simulink model "Vehicle_Model_999_Modular_roll_gradient"  (R2025b)
settings: Solver=ode23tb  StartTime=0.0  StopTime=30  MaxStep=0.001  RelTol=1e-3
values from neighbouring files (symbols this model uses):
  init_r = 0    [Run_this_first.m]
  init_vx = 0    [Run_this_first.m]
  init_vy = 0    [Run_this_first.m]
  Ki_array = zeros(size(Vx_array))    [Torque_vectoring_lookup_table_v3.m]    (also in Torque_vectoring_workspace_lookuptable_v2.m)
  Kp_array = zeros(size(Vx_array))    [Torque_vectoring_workspace_lookuptable_v2.m]
  ku = (lr*m/(cf*(lf+lr))) - (lf*m/(cr*(lf+lr)))    (= -0.000176093739153)    [Torque_vectoring_lookup_table_v3.m]    (also in Torque_vectoring_workspace_lookuptable_v2.m)
  m = Par.m    [LapSim_Endurance_final_ts_v2.m]    (also in Lap_Sim_Final_inverse.m = Par.Mass; Lapsim_Endurance_final_ts.m; New_LapSim_final_ts_v1.m = Par.Mass; Torque_vectoring_lookup_table_v3.m = 270)
  Par = struct()    [Load_vehicle_parameters.m]
  path_Theta = unwrap(atan2(dY, dX))    [New_LapSim_final_ts_v1.m]
  sus_par = struct()    [Load_sus_parameters.m]
  TireData = []    [Lapsim_final_for_app.m]
  V_ref = 45    [Run_this_first.m]
  Vx_array = 1:2:21    [Torque_vectoring_lookup_table_v3.m]    (also in Torque_vectoring_workspace_lookuptable_v2.m = 1:1:21)
undefined symbols (not defined in the file or in its folder): Battery, Brake_Val, ctrl_Brake, ctrl_s, ctrl_Steer, ctrl_Throttle, ctrl_Velocity, HP, Motor, path_X, path_Y, steer_input, Steer_Val, TC_target_slip, Throttle_Val
libraries: simulink x9, autolibshared x3, simulink_extras x2, BatteryEstimators x1
(part 3 of 4)

== matlab function Vehicle_Model_999_Modular_roll_gradient/Vehicle dynamics/Wheel_dynamics/Wheel Dynamics/MATLAB Function ==
  data: T_in input; Omega_dot output; Fx_rr input; Fx_tire input; Omega input; Par parameter
function Omega_dot = fcn(T_in, Fx_rr, Fx_tire, Omega, Par)
%#codegen
    
    % 1. Enforce Column Vectors (Protects against array dimension mismatch)
    T_in = T_in(:);
    Fx_rr = Fx_rr(:);
    Fx_tire = Fx_tire(:);
    Omega = Omega(:);

    % 2. Constants
    R = Par.R0;
    Iw = Par.Iw;
    
    % Rotational damping parameter (fallback to 0.1 if not yet in Par struct)
    % Recommend updating to: b_w = Par.b_w;
    b_w = 0.1; 
    
    % 3. Separate Drive and Brake capacities
    % Note: Assumes T_in > 0 is forward drive, T_in < 0 is braking. 
    T_drive = max(T_in, 0); 
    T_brake_capacity = abs(min(T_in, 0)); 
    
    % Smooth directional multiplier to avoid zero-crossing step discontinuities
    Rotation_Dir = tanh(10 .* Omega);
    
    % 4. Calculate external torques BEFORE brakes are applied
    T_tire_reaction = abs(Fx_rr .* R) .* Rotation_Dir;
    T_tire = Fx_tire .* R;
    T_damping = b_w .* Omega;
    
    % Net torque tending to move the wheel
    T_pre_brake = T_drive - T_tire_reaction - T_tire - T_damping;
    
    % 5. Continuous Blended Brake Logic
    % Dynamic Braking (When Moving): Opposes current rotation
    T_brake_dynamic = -T_brake_capacity .* Rotation_Dir;
    
    % Static Braking (When Stopped): Clamps down to oppose external forces
    % Limits the opposing torque to not exceed available brake capacity
    T_brake_static = -max(min(T_pre_brake, T_brake_capacity), -T_brake_capacity);
    
    % Blend factor: approaches 0 when stopped, approaches 1 when moving
    moving_flag = abs(tanh(10 .* Omega));
    
    % Final applied brake torque
    T_brake_actual = (moving_flag .* T_brake_dynamic) + ((1 - moving_flag) .* T_brake_static);
    
    % 6. Compute Angular Acceleration
    T_net = T_pre_brake + T_brake_actual;
    Omega_dot = T_net ./ Iw;
end

== matlab function Vehicle_Model_999_Modular_roll_gradient/Inputs/MATLAB Function ==
  data: ideal_ref_vel input; y output
function y = fcn(ideal_ref_vel)

y = max(ideal_ref_vel,7);
% y = 1.193*max(ideal_ref_vel,1.5);
% y = 11.461;

== matlab function Vehicle_Model_999_Modular_roll_gradient/E-powertrain/Torque Distribution/MATLAB Function ==
  data: T_wheel input; omega input; T_FL output; T_brake_vec input; T_FR output; T_RL output; T_RR output
function [T_FL, T_FR, T_RL, T_RR] = torque_combiner(T_wheel, omega, T_brake_vec)
%#codegen
    % INPUTS:
    % T_wheel:     4x1 [FL, FR, RL, RR] Motor Torque Request (from Throttle)
    % omega:       4x1 [FL, FR, RL, RR] Wheel Speeds (rad/s)
    % T_brake_vec: 4x1 Brake Capacity (Negative values expected)
    
    % --- 1. INITIALIZATION ---
    T_FL = 0.0; T_FR = 0.0; T_RL = 0.0; T_RR = 0.0;
    
    % PARAMETERS
    w_threshold = 2.0;  % [rad/s] Speed below which we switch to linear damping
    brake_active_threshold = 100.0; % [Nm] Torque to consider "Brakes Active"
    
    % Get absolute brake capacities
    B_FL = abs(T_brake_vec(1));
    B_FR = abs(T_brake_vec(2));
    B_RL = abs(T_brake_vec(3));
    B_RR = abs(T_brake_vec(4));
    
    % --- 2. BRAKE PRIORITY LOGIC (The Fix for Rear Spin) ---
    % If the driver is braking hard, we CUT motor torque.
    % This prevents the "fighting" that causes the rear wheels to spin at 115 rad/s.
    total_brake_force = B_FL + B_FR + B_RL + B_RR;
    
    % Factor: 1.0 = Full Drive, 0.0 = Throttle Cut
    % If braking > threshold, we cut throttle to 0.
    if total_brake_force > brake_active_threshold
        throttle_factor = 0.0; 
    else
        throttle_factor = 1.0;
    end
    
    % Apply the cut to the motor inputs
    T_motor_effective = T_wheel * throttle_factor;
    
    % --- 3. ROBUST BRAKE CALCULATION (Viscous Region) ---
    % This local logic prevents solver crashes when wheels lock (w=0)
    % It uses linear damping near zero speed.
    
    % Fronts (Motor + Brake) - Front motors evaluate to 0
    T_FL = T_motor_effective(1) + apply_brake_physics(omega(1), B_FL, w_threshold);
    T_FR = T_motor_effective(2) + apply_brake_physics(omega(2), B_FR, w_threshold);
    
    % Rears (Motor + Brake)
    T_brake_RL = apply_brake_physics(omega(3), B_RL, w_threshold);
    T_brake_RR = apply_brake_physics(omega(4), B_RR, w_threshold);
    
    % Combine: Effective Motor (Positive) + Braking (Negative)
    T_RL = T_motor_effective(3) + T_brake_RL;
    T_RR = T_motor_effective(4) + T_brake_RR;
end

% --- HELPER LOGIC ---
function T_out = apply_brake_physics(w, Capacity, w_th)
    % If moving fast: Constant Friction (Capacity)
    % If moving slow: Viscous Damping (Linear line to 0)
    if abs(w) < w_th
        % Linear region (Like moving through honey)
        % This forces the torque to exactly 0 as speed hits 0.
        T_out = -Capacity * (w / w_th);
    else
        % Sliding region (Full friction)
        T_out = -Capacity * sign(w);
    end
end

== matlab function Vehicle_Model_999_Modular_roll_gradient/E-powertrain/Torque Distribution/Torque Vectoring/MATLAB Function ==
  data: vectored_torques output; wheel_torques input; yaw_moment input; Par parameter; Motor parameter
function vectored_torques = fcn(wheel_torques,yaw_moment,Par,Motor)
max_wheel_torque = Motor.T_peak_limit * Motor.gear_ratio* Motor.overall_efficiency;
torque_difference = yaw_moment*(Par.R0/(Par.TW));
T_FL = wheel_torques(1);    
T_FR = wheel_torques(2);
T_RL = max(0,min(wheel_torques(3) - (torque_difference),max_wheel_torque));
T_RR = max(0,min(wheel_torques(4) + (torque_difference),max_wheel_torque));

vectored_torques = [T_FL; T_FR; T_RL; T_RR];

== matlab function Vehicle_Model_999_Modular_roll_gradient/E-powertrain/Torque Distribution/Torque Vectoring/PID controller in time domain ==
  settings: updateMethod=DISCRETE
  data: ref input; yaw_moment output; y input; Kp input; Ki input; Par parameter; u_unsat output; error output; Motor parameter
function [yaw_moment,u_unsat,error] = pid_controller(ref, y, Kp, Ki,Par,Motor)
T = Par.TW;
R0 = Par.R0;
Half_T = T/2;


% Custom PI Controller with Clamping Anti-Windup

% Motor torque limits
T_max_motor = Motor.T_peak_limit*Motor.gear_ratio*Motor.overall_efficiency;  
T_min_motor = -T_max_motor;  

% Force limit of each tire:
f_max = T_max_motor/R0;
f_min = T_min_motor/R0;

% Yaw_moment limits
u_max = f_max * Half_T;
u_min = f_min * Half_T;

% Persistent variables
persistent integral prev_error;
if isempty(integral)
    integral = 0;
    prev_error = 0;
end

% Sample time
T = 0.001;

% Compute error
error = ref - y;

% **Proportional Term**
P = Kp * error;

% **Integral Term with Clamping**
I = Ki * integral;

% Compute raw control signal
u_unsat = P + I;

%Clamping Anti-Windup
if u_unsat > u_max
    yaw_moment = u_max;
    % Freeze integral
elseif u_unsat < u_min
    yaw_moment = u_min;
    % Freeze integral
else
    yaw_moment = u_unsat;
    % Update integral only if NOT saturated
    integral = integral + 0.5* T * (error + prev_error);
end

% Store previous error
prev_error = error;
end

== matlab function Vehicle_Model_999_Modular_roll_gradient/E-powertrain/Torque Distribution/Torque Vectoring/Target yaw rate/MATLAB Function ==
  data: vx input; target_yaw output; delta input; Dy input; Fz input; Par parameter; ideal_yaw output; ku parameter; tv_enable output
function [target_yaw, ideal_yaw, tv_enable] = target_yaw_rate(vx, delta, Dy, Fz, Par, ku)
    % Prevent division by zero
    epsilon = 0.01;                                                                                 
    
    % Always calculate the natural ideal yaw rate
    ideal_yaw = (delta * vx) / ((vx^2 * ku) + (Par.Lf + Par.Lr));                                     
    
    % Deadzone logic: Check if we are outside the deadzone
    if abs(delta) > deg2rad(8) && vx > 1
        % Condition met: Turn ON torque vectoring
        tv_enable = true; 
        
        mu_array = Dy ./ Fz;                                                                            
        avg_rear_mu = mean(mu_array(3:4));   
        yaw_limit = (avg_rear_mu * Par.g) / (vx + epsilon);                                                    
        
        % Clamp to physical limits
        if ideal_yaw < -yaw_limit 
            target_yaw = -yaw_limit;
        elseif ideal_yaw > yaw_limit
            target_yaw = yaw_limit;
        else 
            target_yaw = ideal_yaw;
        end
        
    else
        % Condition NOT met: Turn OFF torque vectoring
        tv_enable = false; 
        
        % Crucial: Still output the natural yaw rate so the error is zero 
        % when the controller turns back on, preventing sudden spikes.
        target_yaw = ideal_yaw; 
    end
end

== matlab function Vehicle_Model_999_Modular_roll_gradient/Vehicle dynamics/Suspension/Toe_calculation/toe_fl1 ==
  data: Fy_tire input size=[4 1]; Fx_tire input size=[4 1]; Toe_fl output; Mz input size=[4 1]; sus_par parameter; Toe_fr output; Toe_rl output; Toe_rr output
function [Toe_fl,Toe_fr,Toe_rl,Toe_rr] = fcn(Fy_tire,Fx_tire,Mz,sus_par)

Toe_fl = -sus_par.Toe_f_static + sus_par.C_Fx_toe*Fx_tire(1) + sus_par.C_Fy_toe*Fy_tire(1) + sus_par.C_Mz_toe*Mz(1);

Toe_fr = sus_par.Toe_f_static + sus_par.C_Fx_toe*Fx_tire(2) +sus_par.C_Fy_toe*Fy_tire(2) + sus_par.C_Mz_toe*Mz(2);

Toe_rl = -sus_par.Toe_r_static + sus_par.C_Fx_toe*Fx_tire(3) +sus_par.C_Fy_toe*Fy_tire(3) + sus_par.C_Mz_toe*Mz(3);

Toe_rr = sus_par.Toe_r_static + sus_par.C_Fx_toe*Fx_tire(4) +sus_par.C_Fy_toe*Fy_tire(4) + sus_par.C_Mz_toe*Mz(4);

== matlab function Vehicle_Model_999_Modular_roll_gradient/E-powertrain/Torque Distribution/Traction Control/MATLAB Function1 ==
  settings: updateMethod=DISCRETE
  data: lambda_ref input; lambda_actual input size=[4 1]; throttle_cmd output; Kp input; Ki input; Kd input; Motor parameter
function throttle_cmd = pid_traction_controller(lambda_ref, lambda_actual, Kp, Ki, Kd, Motor)
%#codegen

% Fixed time step
dt = 0.001;

% Persistent states initialized as 4x1 vectors for 4 wheels
% Assuming standard ordering: [Front-Left; Front-Right; Rear-Left; Rear-Right]
persistent integrator prev_error;
if isempty(integrator)
    integrator = zeros(4, 1);
end
if isempty(prev_error)
    prev_error = zeros(4, 1);
end

% Ensure inputs are column vectors for consistent matrix operations
lambda_actual = lambda_actual(:); 

% ── 1. Error ───────────────────────────────────────
% Calculates error for all 4 wheels simultaneously
e = lambda_ref - lambda_actual;

% ── 2. Derivative (rate of slip change) ────────────
de = (e - prev_error) / dt;

% ── 3. Conditional Integration (ANTI-WINDUP) ───────
% Create a binary mask (1 where true, 0 where false) for the windup condition
integration_mask = abs(e) < 0.2; 

% Multiply by the mask to only integrate the wheels that meet the condition
integrator = integrator + (e .* integration_mask) * dt;

% Clamp integrator bounds for all 4 wheels
integrator = max(min(integrator, 0.5), -0.5);

% ── 4. PID Output ──────────────────────────────────
% Using element-wise multiplication (.*) allows Kp, Ki, Kd to be either 
% scalars (applied to all wheels) or 4x1 vectors (individual gains per wheel)
throttle_pid = Kp .* e + Ki .* integrator + Kd .* de;

% ── 5. Clamp output ────────────────────────────────
% Clamps the PID output between 0.0 and 1.0 for all wheels
throttle_pid = max(min(throttle_pid, 1.0), 0.0);

% ── 6. Traction control logic ──────────────────────
% Calculate final torque commands for all wheels
throttle_cmd = throttle_pid * Motor.T_peak_limit * Motor.gear_ratio;

% ── 7. RWD Constraint ──────────────────────────────
% Force the front wheels (indices 1 and 2) to output 0 torque
throttle_cmd(1:2) = 0;

% ── 8. Store previous error ────────────────────────
prev_error = e;

end

== matlab function Vehicle_Model_999_Modular_roll_gradient/E-powertrain/Battery Pack/MATLAB Function ==
  data: Voc_pack input; v_bus output; R0_pack input; V_rc input; I_dc input
function v_bus = fcn(Voc_pack, R0_pack, V_rc, I_dc)
    % This function calculates the terminal voltage of the battery pack.
    % Voc_pack: Output from OCV LUT multiplied by Ns
    % R0_pack:  Output from R0 LUT multiplied by (Ns/Np)
    % V_rc:     Instantaneous voltage across the RC branch
    % I_dc:     Total DC current from the motor

    % 1. Calculate the instantaneous Ohmic drop (Ohm's Law)
    V_ohmic = I_dc * R0_pack;

    % 2. Calculate terminal voltage (Vt = Voc - V_ohmic - V_rc)
    v_bus = Voc_pack - V_ohmic - V_rc;

    % 3. Safety: Ensure voltage doesn't drop below a physical floor (e.g., 2.5V * Ns)
    % This prevents simulation crashes if the battery is fully depleted.
    % v_bus = max(v_bus, 2.5 * 144); 
end

== matlab function Vehicle_Model_999_Modular_roll_gradient/Inputs/steer_input_simulink/MATLAB Function1 ==
  data: delta output; Par parameter; ku parameter
function delta = fcn(Par,ku)

psi_dot = 2*pi/5;   % yaw rate in rad/s for 5 sec skidpad
vx = 11.461; % Velocity tangent to the circle 
ku = ku;
delta = Par.WB*(psi_dot/vx)+ku*vx*psi_dot;

== matlab function Vehicle_Model_999_Modular_roll_gradient/Vehicle dynamics/Rolling and Drag forces/Aero Drag ==
  data: vx input; B_F_aero output; vy input; aero_par parameter
function B_F_aero = fcn(vx, vy, aero_par)

    %#codegen
    % AERODYNAMIC DRAG (Body Frame)
    % Calculates drag vector acting on the CG.
%
% Inputs:
%   vx, vy : Vehicle Velocities in Body Frame [m/s]
%   Par    : Parameters (.Cd, .Area, .rho, .C_side)
%
% Output:
%   B_F_aero : [Fx; Fy; 0] Aerodynamic Force Vector [N]

    % 1. Longitudinal Drag (Standard)
    % Fx = -0.5 * rho * Cd * Area * vx^2
    % Usage: sign(vx) ensures drag always opposes motion
    Fx_drag = 0.5 * aero_par.rho * aero_par.Cd * aero_par.Area * vx * abs(vx);

    % 2. Lateral Drag (Side Force) - Optional
    % Only relevant if sliding significantly.
    % If Par.C_side is not defined, calculate as 0.
    if isfield(aero_par, 'C_side') && aero_par.C_side > 0
        % Side area is often approx same as Frontal Area or larger
        % Fy = - 0.5 * rho * C_side * Area_Side * vy^2
        Fy_drag = -0.5 * aero_par.rho * aero_par.C_side * aero_par.Area * vy * abs(vy);
    else
        Fy_drag = 0;
    end
    
    % 3. Output Vector for Equilibrium Block
    B_F_aero = [Fx_drag; Fy_drag; 0];

end

== matlab function Vehicle_Model_999_Modular_roll_gradient/Vehicle dynamics/Brakes/MATLAB Function ==
  data: brake_pedal input; T_brakes output; omega input; Brake parameter; T_mag_Front output; T_mag_Rear output
function [T_brakes,T_mag_Front,T_mag_Rear]  = fcn(brake_pedal, omega, Brake)
    % BRAKE TORQUE CALCULATION
    % Converts normalized pedal/actuator position into physical torque
    % and ensures torque direction opposes wheel rotation.
    
    % 1. Calculate Magnitude of Torque based on Command (0-1)
    % We use the static max targets from the design sheet
    T_mag_Front = brake_pedal * Brake.MaxTorque_Wheel_F;
    T_mag_Rear  = brake_pedal * Brake.MaxTorque_Wheel_R;
    
    % Initialize output vector (FL, FR, RL, RR)
    T_brakes = zeros(4, 1);
    
    % 2. Apply Torque per Wheel with Directional Logic
    % Loop through all 4 wheels to apply logic individually
    % Indices: 1=FL, 2=FR, 3=RL, 4=RR
    
    for i = 1:4
        % Determine if this is a Front (1,2) or Rear (3,4) wheel
        if i <= 2
            T_req = T_mag_Front;
        else
            T_req = T_mag_Rear;
        end
        
        % Directional Check:
        % Torque must be negative if omega is positive, and vice versa.
        % -sign(omega) flips the torque direction.
        T_applied = T_req * -sign(omega(i));
        
        % Zero-Speed Cutoff:
        % If wheel is nearly stopped, clamp torque to zero to prevent 
        % the simulation from "driving" the car backwards.
        % if abs(omega(i)) < Brake.ZeroSpeedThreshold
        %     T_applied = 0;
        % 
            % Advanced: Ideally, below threshold, T_brake should act as 
            % a viscous damper or Coulomb friction that exactly cancels 
            % remaining motion, but zeroing is sufficient for laptime sims.
        % end
        
        T_brakes(i) = T_applied;
    end
end

== matlab function Vehicle_Model_999_Modular_roll_gradient/Vehicle dynamics/Rolling and Drag forces/MATLAB Function ==
  data: u input; y output
function y = fcn(u)

y = u(1);

== matlab function Vehicle_Model_999_Modular_roll_gradient/Vehicle dynamics/Rolling and Drag forces/Rolling Forces ==
  data: Fz input; Fx_rr_b output; Steer_FL input; Steer_FR input; Fy_rr_b output; Par parameter
function [Fx_rr_b, Fy_rr_b] = fcn(Fz, Steer_FL, Steer_FR, Par)

    %#codegen

    % 1. Setup
    C_rr = Par.C_rr; 
    
    % Construct Steering Vector (Assuming Rear Steer = 0)
    Delta = [Steer_FL; Steer_FR; 0; 0];

    % Initialize Outputs
    Fx_rr_b = zeros(4, 1);
    Fy_rr_b = zeros(4, 1);

    % 2. Calculate & Resolve Forces (Vectorized Loop)
    for i = 1:4
        
        % Magnitude (Always positive Fz)
        F_mag = C_rr * abs(Fz(i));
        
        % B. Define Force Vector in Wheel Frame
        F_xw = - F_mag;
        F_yw = 0;
        
        % C. Transform to Body Frame (Rotation)
        d = Delta(i);
        c = cos(d);
        s = sin(d);
        
        % Rotate: F_body = Rz(delta) * F_wheel
        % Fx_b = Fx_w*cos - Fy_w*sin
        Fx_rr_b(i) = F_xw * c - F_yw * s;
        
        % Fy_b = Fx_w*sin + Fy_w*cos
        Fy_rr_b(i) = F_xw * s + F_yw * c;
    end

end

== matlab function Vehicle_Model_999_Modular_roll_gradient/Vehicle dynamics/Force and Torque Equilibrium/Force and Torque Equilibrium ==
  data: B_Fx input; ax output size=1; ay output size=1; B_Fy input; B_Fx_roll input; B_Fy_roll input; B_F_drag input; yawrate input; vx input; vy input; r_dot output size=1; Par parameter; ay_sensor output; ax_sensor output; Mz_individual output
function [ax, ay, r_dot, ay_sensor, ax_sensor,Mz_individual] = fcn(B_Fx, B_Fy, B_Fx_roll, B_Fy_roll, B_F_drag, yawrate, vx, vy, Par)
%#codegen

    % 1. Enforce Column Vectors 
    % (Protects against dimension mismatch if an input is accidentally 1x4)
    B_Fx = B_Fx(:);
    B_Fy = B_Fy(:);
    B_Fx_roll = B_Fx_roll(:);
    B_Fy_roll = B_Fy_roll(:);
    
    % 2. Geometry Setup
    m = Par.m;
    Iz = Par.Iz;
    
    % Create Geometry Vectors for [FL; FR; RL; RR]
    % x_arms: Distance from CG to axle (Positive = Front)
    x_arms = [Par.Lf;   Par.Lf;  -Par.Lr;  -Par.Lr];
    
    % y_arms: Distance from centerline (Positive = Left)
    t = Par.TW / 2;
    y_arms = [ t;      -t;        t;      -t];
    
    % 3. Total Corner Forces
    Fx_total = B_Fx + B_Fx_roll; 
    Fy_total = B_Fy + B_Fy_roll; 
    
    % 4. Linear Force Equilibrium
    Sigma_Fx = sum(Fx_total) - B_F_drag(1);
    Sigma_Fy = sum(Fy_total) - B_F_drag(2);
    
    % 5. Linear Accelerations 
    ax = (Sigma_Fx / m) + (vy * yawrate);
    ay = (Sigma_Fy / m) - (vx * yawrate);
    
    ax_sensor = Sigma_Fx / m;
    ay_sensor = Sigma_Fy / m;
    
    % 6. Moment Equilibrium (Vectorized)
    Mz_individual = (x_arms .* Fy_total) - (y_arms .* Fx_total);
    Sigma_Mz = sum(Mz_individual);
    
    % 7. Yaw Acceleration (rad/s^2)
    r_dot = Sigma_Mz / Iz;
end

== matlab function Vehicle_Model_999_Modular_roll_gradient/Vehicle dynamics/Fx, Fy calculations with grip limit/Simplified Tire Model ==
  data: Fz input; Fx output size=4; slip_ratios input; slip_angles input; camber_angles input; Fy output size=4; Self_aligning_torque output size=4; Mu_x output size=4; Mu_y output size=4; Dx output; TireData parameter; Par parameter; sus_par parameter; Dy output size=[4 1]
function [Fx, Fy, Self_aligning_torque, Mu_x, Mu_y,Dx, Dy] = fcn(Fz, slip_ratios, slip_angles, camber_angles, TireData, Par, sus_par)
%#codegen
% =========================================================================
%  VECTORIZED MAGIC FORMULA 5.2 (4-WHEEL)
% =========================================================================

    % 0. Enforce Column Vectors (Crash Protection)
    Fz = Fz(:);
    slip_ratios = slip_ratios(:);
    slip_angles = slip_angles(:);
    camber_angles = camber_angles(:);

    % 1. EXTRACT PARAMETERS (Scalars)
    p = TireData;
    s = TireData.Scales;
    Fz0 = p.FNOMIN;
    R0  = p.R0;
    par = Par;
    
    % 2. INPUT SAFETY & NORMALIZATION
    % Clamp negative loads to 0 (Tires can't pull ground)
    Fz_safe = max(Fz, 0); 
    
    % Avoid division by zero for Mu calculations later
    Fz_denom = max(Fz_safe, 1.0); 
    
    % Normalized Load (dfz) - Vectorized
    dfz = (Fz_safe - Fz0) ./ Fz0;
    
    % ---------------------------------------------------------------------
    % A. LONGITUDINAL FORCE (Fx) - VECTORIZED
    % ---------------------------------------------------------------------
    Cx = p.PCX1 * s.LCX;
    
    % Friction Coeff Mu_x
    mu_x_base = (p.PDX1 + p.PDX2 .* dfz) .* (1 - p.PDX3 .* camber_angles.^2) .* s.LMUX;
    Dx = mu_x_base .* Fz_safe;
    
    % Stiffness Kx
    Kx = Fz_safe .* (p.PKX1 + p.PKX2 .* dfz) .* exp(p.PKX3 .* dfz) .* s.LKX;
    
    % Stiffness Factor Bx
    Bx = Kx ./ (Cx .* Dx + 1e-6); 
    
    % Shifts (Horizontal & Vertical)
    Shx = (p.PHX1 + p.PHX2 .* dfz) .* s.LHX;
    Svx = Fz_safe .* (p.PVX1 + p.PVX2 .* dfz) .* s.LVX;
    
    % Composite Slip
    k_s = slip_ratios + Shx;
    
    % Curvature Ex (Sign Dependent)
    Ex = (p.PEX1 + p.PEX2 .* dfz + p.PEX3 .* dfz.^2) .* (1 - p.PEX4 .* sign(k_s)) .* s.LEX;
    Ex(Ex > 1) = 1; % Clamp
    
    % Calculation
    Bx_k = Bx .* k_s;
    Fx = Dx .* sin(Cx .* atan(Bx_k - Ex .* (Bx_k - atan(Bx_k)))) + Svx;
    
    % ---------------------------------------------------------------------
    % B. LATERAL FORCE (Fy) - VECTORIZED
    % ---------------------------------------------------------------------
    Cy = p.PCY1 * s.LCY;
    
    % Friction Coeff Mu_y
    mu_y_base = (p.PDY1 + p.PDY2 .* dfz) .* (1 - p.PDY3 .* camber_angles.^2) .* s.LMUY;
    Dy = mu_y_base .* Fz_safe;
    
    % Cornering Stiffness Ky (Trig Form)
    Ky = p.PKY1 .* Fz0 .* sin(2 .* atan(Fz_safe ./ (p.PKY2 .* Fz0))) .* (1 - p.PKY3 .* abs(camber_angles)) .* s.LKY;
    
    % Poly fallback check (if PKY2 implies poly form)
    if (Ky(1) < 1)
        Ky = Fz_safe .* (p.PKY1 + p.PKY2 .* dfz) .* s.LKY;
    end
    
    By = Ky ./ (Cy .* Dy + 1e-6);
    
    % Shifts 
    Shy = (p.PHY1 + p.PHY2 .* dfz) .* s.LHY;
    Svy = Fz_safe .* (p.PVY1 + p.PVY2 .* dfz) .* s.LVY;
    
    % FIXED: Removed the 0* debug multiplier
    a_s = slip_angles + Shy;
    
    % Curvature Ey (Sign Dependent)
    Ey = (p.PEY1 + p.PEY2 .* dfz) .* (1 - (p.PEY3 + p.PEY4 .* camber_angles) .* sign(a_s)) .* s.LEY;
    Ey(Ey > 1) = 1;
    
    % Calculation
    By_a = By .* a_s;
    % FIXED: Removed the 0* debug multiplier
    Fy = -(Dy .* sin(Cy .* atan(By_a - Ey .* (By_a - atan(By_a)))) + Svy);
    
    % ---------------------------------------------------------------------
    % C. SELF-ALIGNING TORQUE (Mz) - VECTORIZED
    % ---------------------------------------------------------------------
    % Peak Trail Dt
    Dt = (p.QDZ1 + p.QDZ2 .* dfz) .* (1 - p.QDZ3 .* abs(camber_angles)) .* R0 .* s.LTR;
    
    % Trail Slope Bt
    Bt = (p.QBZ1 + p.QBZ2 .* dfz + p.QBZ3 .* dfz.^2) .* (1 + p.QBZ4 .* abs(camber_angles)) .* (s.LKY / s.LMUY);
    
    Ct = p.QCZ1; % Scalar
    Et = (p.QEZ1 + p.QEZ2 .* dfz + p.QEZ3 .* dfz.^2);
    
    % Trail 't' Calculation(Pneumatic trail)
    Bt_a = Bt .* a_s;
    alpha_t = Bt_a - Et .* (Bt_a - atan(Bt_a));
    t = Dt .* cos(Ct .* atan(alpha_t)) .* cos(a_s);
    
    % Trail 'tm' Calculation(mechanical trail)
    tm = par.R0 .* tan(sus_par.Caster_static);
    
    % Residual Mzr
    Dr = Fz_safe .* R0 .* (p.QDZ6 + p.QDZ7 .* dfz) .* s.LRES;
    Br = 10;
    Mzr = Dr .* cos(atan(Br .* a_s));
    
    % Final Mz (Standard Restoring: Negative Slope)
    Self_aligning_torque = -(t + tm) .* Fy + Mzr;
    
    % ---------------------------------------------------------------------
    % D. OUTPUTS 
    % ---------------------------------------------------------------------
    % Friction Coeffs
    Mu_x = Fx ./ Fz_denom;
    Mu_y = Fy ./ Fz_denom;
    % theta = atan(Fx./Fy);
    % Fx_tire_new = min(Fx,Dx.*sin(theta));
    % Fy_tire_new = min(Fy,Dy.*cos(theta));
    % Note on Lifted Wheels: Because Fz_safe mathematically zeroes out 
    % Dx, Kx, Dy, Ky, Dt, and Dr, the outputs smoothly evaluate to 0 
    % without needing the commented-out boolean masking. 
    % This is faster and safer for C-code generation.
end

== matlab function Vehicle_Model_999_Modular_roll_gradient/E-powertrain/Torque Distribution/Traction Control/MATLAB Function2 ==
  data: TC_output output; torque_pid input; torque_wheel input
function TC_output = fcn(torque_pid, torque_wheel)
% Initialize TC_output
TC_output = zeros(4,1);

for i = 1:4

    if torque_pid(i) < torque_wheel(i)
        TC_output(i) = torque_pid(i);
    else
        TC_output(i) = torque_wheel(i);
    end
end

== matlab function Vehicle_Model_999_Modular_roll_gradient/E-powertrain/Motor/Motor with Field Weakening ==
  data: kt input; rpm_4x1 input; Torque_Nm_vec output; throttle_scalar input; v_dc_bus input; Motor parameter; I_dc_total output size=[1]; P_total_sum output size=[1]
function [Torque_Nm_vec, I_dc_total,P_total_sum] = fcn(kt, rpm_4x1, throttle_scalar, v_dc_bus, Motor)
    % Inputs:
    %   rpm_4x1         : [FL; FR; RL; RR] wheel speeds in RPM
    %   throttle_scalar : Driver input (0 to 1)
    %   v_dc_bus        : Battery voltage (V)
    %   Motor           : Struct containing constants
    
    % --- 1. Distribute Inputs ---
    % We apply the same throttle to both motors for now.
    % We extract the Rear-Left (index 3) and Rear-Right (index 4) speeds.
    rpm_targets = [rpm_4x1(3); rpm_4x1(4)]; 
    throttle_vec = [throttle_scalar; throttle_scalar];
    psi_m = kt / (1.5 * Motor.p * sqrt(2)); 

    % Initialize storage
    Torque_Nm_vec = zeros(2, 1); % [T_RL; T_RR]
    P_elec_vec = zeros(2, 1);
    
    for i = 1:2
        % --- 2. Redline & Mechanical Limit Check ---
        if abs(rpm_targets(i)) >= Motor.n_max
            continue; % Torque and Power remain 0
        end

        % --- 3. Electrical Conversions ---
        omega_m = rpm_targets(i) * (2*pi/60);
        omega_e = max(abs(omega_m * Motor.p), 0.1); 
        V_max_phase = v_dc_bus / sqrt(3);
        I_cmd_peak = Motor.I_max_rms * sqrt(2) * throttle_vec(i);

        % --- 4. Region Selection: MTPA vs Field Weakening ---
        V_req_mtpa = omega_e * sqrt((Motor.L * I_cmd_peak)^2 + psi_m^2);
        
        if V_req_mtpa <= V_max_phase
            id = 0;
            iq = I_cmd_peak;
        else
            % Field Weakening logic for Fischer Motor
            a = Motor.L^2;
            b = 2 * Motor.L * psi_m;
            c = Motor.psi_m^2 + (Motor.L * I_cmd_peak)^2 - (V_max_phase / omega_e)^2;
            
            id = (-b + sqrt(max(0, b^2 - 4 * a * c))) / (2 * a);
            id = max(min(id, 0), -I_cmd_peak); 
            iq = sqrt(max(0, I_cmd_peak^2 - id^2));
        end

        % --- 5. Torque and Power Calculation ---
        T_gen = 1.5 * Motor.p * psi_m * iq;
        Torque_Nm_vec(i) = min(T_gen, Motor.T_peak_limit);

        % P_elec = P_mechanical + P_copper_losses
        P_mech = abs(Torque_Nm_vec(i) * omega_m);
        P_copper = 3 * 0.126 * (I_cmd_peak / sqrt(2))^2;
        P_elec_vec(i) = P_mech + P_copper;
    end

    % --- 6. Battery Summation ---
    P_total_sum = sum(P_elec_vec);
    if v_dc_bus > 20
        % Calculate total current draw for the Molicel P45B pack
        I_dc_total = P_total_sum / (0.95 * v_dc_bus);

    else
        I_dc_total = 0;
    end
end

== matlab function Vehicle_Model_999_Modular_roll_gradient/Drivetrain/Thermal/MATLAB Function ==
  settings: updateMethod=DISCRETE  sampleTime=1
  data: Q_total output size=1; I_rms input; Speed_RPM input; P_iron_rotor input; T_motor_K input; T_motor_C output; R_actual output; kt_actual output
function [Q_total, T_motor_C, R_actual, kt_actual] = motor_thermal_logic(I_rms, Speed_RPM, P_iron_rotor, T_motor_K)
    %#codegen
    
    %% 1. Force outputs to be SCALAR doubles
    % This stops the "variable-size matrix" error
    Q_total   = double(0); 
    T_motor_C = double(0);
    R_actual  = double(0);
    kt_actual = double(0);

    %% 2. Constants from Fischer Datasheet
    R_ref   = 0.126;    % Phase resistance at 20°C
    kt_ref  = 0.492;    % Torque constant
    alpha   = 0.00393;  % Temp coefficient for Copper
    gamma_m = 0.001;    % Magnet flux fade (0.1% per degC)
    
    %% 3. Unit Conversion & Calculations
    T_kelvin = double(T_motor_K(1));
    T_motor_C = T_motor_K - 273.15; % Kelvin to Celsius
    
    % Ensure T_motor_C doesn't cause math errors if feedback is zero at start
    R_actual = R_ref * (1 + alpha * (T_motor_C - 20)); 
    kt_actual = kt_ref * (1 - gamma_m * (T_motor_C - 20)); 
    
    % Force I_rms to be treated as a single scalar value
    I_val = double(I_rms(1));
    P_cu = 3 * (I_val^2) * R_actual; 
    
    % Final sum forced to scalar double
    Q_total = P_cu + double(P_iron_rotor(1)); 
end

== matlab function Vehicle_Model_999_Modular_roll_gradient/Vehicle dynamics/Suspension/MATLAB Function ==
  data: Z input size=[4 1]; ax input; z_dot output size=[4 1]; ay input; Fz output size=[4 1]; sus_par parameter; Par parameter; TireData parameter; aerodynamic_downforce input
function [z_dot, Fz] = suspension_calculations(Z, ax, ay, sus_par, Par, TireData, aerodynamic_downforce)
    % Extract parameters
    ks_f = sus_par.Ks_f;
    ks_r = sus_par.Ks_r;
    mr_f = sus_par.Motion_ratio_f;
    mr_r = sus_par.Motion_ratio_r;
    kt = TireData.VERTICAL_STIFFNESS;
    m = Par.m;
    g = 9.81;
    T = Par.TW;
    WD_f = Par.WD_f;
    WD_r = Par.WD_r;
    hcgrc = Par.CG_h - Par.RC_h;
    a = 0.51;
    b = 0.49;
    L = Par.WB;
    k_damp_f = sus_par.C_damp_f;
    k_damp_r = sus_par.C_damp_r;
    k_arb_f = sus_par.K_arb_f;
    k_arb_r = sus_par.K_arb_r;
    zr_f = sus_par.RC_h_f;
    zr_r = sus_par.RC_h_r;

    % Ensure inputs are row vectors to support time-series vectorization
    ax = ax(:)'; 
    ay = ay(:)';
    aerodynamic_downforce = aerodynamic_downforce(1:1)'; % Ensure aero is 1xN

    if size(Z, 1) ~= 4
        Z = Z'; % Force z_dot to be 4xN
    end
    z_fl = Z(1);z_fr = Z(2); z_rl = Z(3); z_rr = Z(4); 
    constant_vetical_load = (Par.sprung_mass + aerodynamic_downforce/g);
    % --- 1. Static & Aero Load Calculation ---
    % Calculates equivalent static weight and distributes downforce. 
    % Results in 4xN arrays if aerodynamic_downforce varies over time.
    Fz_static_fl = (constant_vetical_load*WD_f/2 + Par.unsprung_mass(1))*g;
    Fz_static_fr = (constant_vetical_load*WD_f/2 + Par.unsprung_mass(2))*g;
    Fz_static_rl = (constant_vetical_load*WD_r/2 + Par.unsprung_mass(3))*g;
    Fz_static_rr = (constant_vetical_load*WD_r/2 + Par.unsprung_mass(4))*g;
    
    Fz_static = [Fz_static_fl;
                 Fz_static_fr;
                 Fz_static_rl;
                 Fz_static_rr];

    
    % Wheel rate calculations
    kw_f = ks_f * mr_f^2;
    kw_r = ks_r * mr_r^2;

    % Ride rate calculations
    kr_f = kw_f * kt / (kw_f + kt);
    kr_r = kw_r * kt / (kw_r + kt);

    % Roll rate calculations
    K_phi_f = (kr_f*T^2)/2 + k_arb_f;
    K_phi_r = (kr_r*T^2)/2 + k_arb_r;
    K_phi_total = K_phi_f + K_phi_r;
    % Load Transfer Calculations
    LT_fx = m * ax * hcgrc / L;
    LT_fy_f = (m * ay / T)*( hcgrc*K_phi_f/K_phi_total + b*zr_f/L);
    LT_fy_r = (m * ay / T)*( hcgrc*K_phi_r/K_phi_total + a*zr_r/L);

    % Vectorized Load Transfer (Results in a 4xN Matrix)
    LT = [-LT_fx - LT_fy_f;
          -LT_fx + LT_fy_f;
           LT_fx - LT_fy_r;
           LT_fx + LT_fy_r];

    % --- 4. Normal Load (Fz) ---
    % Combines Static, Aero, and Dynamic Load Transfer
    Fz = Fz_static + LT;
    
    % Wheel vertical velocities (extract rows)
    % z_dot = zeros(4, length(ax)); % Pre-allocate for speed

    z_dot_fl = (LT(1) + aerodynamic_downforce*WD_f/2 - z_fl*(kw_f) - (z_fl - z_fr)*k_arb_f*2/T)/k_damp_f;
    z_dot_fr = (LT(2) + aerodynamic_downforce*WD_f/2 - z_fr*(kw_f) + (z_fl - z_fr)*k_arb_f*2/T)/k_damp_f;
    z_dot_rl = (LT(3) + aerodynamic_downforce*WD_r/2 - z_rl*(kw_r) - (z_rl - z_rr)*k_arb_r*2/T)/k_damp_r;
    z_dot_rr = (LT(4) + aerodynamic_downforce*WD_r/2 - z_rr*(kw_r) + (z_rl - z_rr)*k_arb_r*2/T)/k_damp_r;
    
    z_dot = [z_dot_fl; z_dot_fr; z_dot_rl; z_dot_rr];
end

== matlab function Vehicle_Model_999_Modular_roll_gradient/Vehicle dynamics/Suspension/Roll and pitch angle calculations/Pitch_angle_calcualtions ==
  data: z_wheel input size=[4 1]; Pitch_angle output; Par parameter
function Pitch_angle = fcn(z_wheel,Par)

WB = Par.WB;

% Avg disp calculation per axle 
z_avg_f = (z_wheel(1) + z_wheel(2))/2;
z_avg_r = (z_wheel(3) + z_wheel(4))/2;

Pitch_angle = (z_avg_r- z_avg_f)/WB;

== matlab function Vehicle_Model_999_Modular_roll_gradient/Vehicle dynamics/Suspension/Roll and pitch angle calculations/Roll_angle_calulations ==
  data: z_wheel input size=[4 1]; Roll_angle output; Par parameter
function Roll_angle = fcn(z_wheel,Par)

TW = Par.TW;

% Avg disp calculation per track
z_avg_l = (z_wheel(1) + z_wheel(3))/2;
z_avg_r = (z_wheel(2) + z_wheel(4))/2;

Roll_angle = (z_avg_l - z_avg_r)/TW;

== matlab function Vehicle_Model_999_Modular_roll_gradient/Vehicle dynamics/Force and Torque Equilibrium/MATLAB Function ==
  data: vx input; V_X output; vy input; psi input; V_Y output
function [V_X, V_Y] = Local_To_Global(vx, vy, psi)
    % Rotate local velocities into global velocities
    V_X = (vx * cos(psi)) - (vy * sin(psi));
    V_Y = (vx * sin(psi)) + (vy * cos(psi));
end

== matlab function Vehicle_Model_999_Modular_roll_gradient/Vehicle dynamics/Suspension/MATLAB Function2 ==
  data: Z_dyn input; Camber output; Camber_gain output; HP parameter; sus_par parameter
function [Camber, Camber_gain] = DynamicCamber_FromHP_Zmeters(Z_dyn, HP, sus_par)
%#codegen
% Z_dyn : dynamic wheel vertical displacement from static ride height (meters, + = bump)
% Output Camber [4x1] radians (dynamic absolute camber)

% 1. Configured static camber
static_camber_4x1 = sus_par.Camber_static .* ones(4,1);

% 2. Dynamic displacements in mm (FL, FR, RL, RR)
zw = Z_dyn .* [sus_par.Motion_ratio_f; sus_par.Motion_ratio_f; ...
               sus_par.Motion_ratio_r; sus_par.Motion_ratio_r] .* 1000;

% 3. Extract and Vectorize Hardpoints (Applying side mirroring directly)
% Inner Pivots (Y and Z) - Average of F and R legs to establish the inner pivot axis
UiY = [ (HP.Front.UCA_F(2) + HP.Front.UCA_R(2))*0.5;
       -(HP.Front.UCA_F(2) + HP.Front.UCA_R(2))*0.5;
        (HP.Rear.UCA_F(2)  + HP.Rear.UCA_R(2))*0.5;
       -(HP.Rear.UCA_F(2)  + HP.Rear.UCA_R(2))*0.5 ];

UiZ = [ (HP.Front.UCA_F(3) + HP.Front.UCA_R(3))*0.5;
        (HP.Front.UCA_F(3) + HP.Front.UCA_R(3))*0.5;
        (HP.Rear.UCA_F(3)  + HP.Rear.UCA_R(3))*0.5;
        (HP.Rear.UCA_F(3)  + HP.Rear.UCA_R(3))*0.5 ];

LiY = [ (HP.Front.LCA_F(2) + HP.Front.LCA_R(2))*0.5;
       -(HP.Front.LCA_F(2) + HP.Front.LCA_R(2))*0.5;
        (HP.Rear.LCA_F(2)  + HP.Rear.LCA_R(2))*0.5;
       -(HP.Rear.LCA_F(2)  + HP.Rear.LCA_R(2))*0.5 ];

LiZ = [ (HP.Front.LCA_F(3) + HP.Front.LCA_R(3))*0.5;
        (HP.Front.LCA_F(3) + HP.Front.LCA_R(3))*0.5;
        (HP.Rear.LCA_F(3)  + HP.Rear.LCA_R(3))*0.5;
        (HP.Rear.LCA_F(3)  + HP.Rear.LCA_R(3))*0.5 ];

% Outer Pivots (Y and Z base static values)
UO_Y = [HP.Front.UCA_O(2); -HP.Front.UCA_O(2); HP.Rear.UCA_O(2); -HP.Rear.UCA_O(2)];
LO_Y = [HP.Front.LCA_O(2); -HP.Front.LCA_O(2); HP.Rear.LCA_O(2); -HP.Rear.LCA_O(2)];
TCP_Y = [HP.Front.TCP(2);  -HP.Front.TCP(2);  HP.Rear.TCP(2);  -HP.Rear.TCP(2)];

UO_Z_base  = [HP.Front.UCA_O(3); HP.Front.UCA_O(3); HP.Rear.UCA_O(3); HP.Rear.UCA_O(3)];
LO_Z_base  = [HP.Front.LCA_O(3); HP.Front.LCA_O(3); HP.Rear.LCA_O(3); HP.Rear.LCA_O(3)];
TCP_Z_base = [HP.Front.TCP(3);   HP.Front.TCP(3);   HP.Rear.TCP(3);   HP.Rear.TCP(3)];

% 4. Compute Kinematics Vectorized (All 4 corners at once)
% Dynamic geometry
Camber_d = compute_corner_kinematics(zw, UiY, UiZ, LiY, LiZ, UO_Y, LO_Y, TCP_Y, UO_Z_base, LO_Z_base, TCP_Z_base);

% Static geometry (0 mm travel)
Camber_s_raw = compute_corner_kinematics([0;0;0;0], UiY, UiZ, LiY, LiZ, UO_Y, LO_Y, TCP_Y, UO_Z_base, LO_Z_base, TCP_Z_base);
Camber_s = abs(Camber_s_raw); % Mirroring your original solveCorner_theta logic

% 5. Calculate Deltas (Preserving your exact original quadrant/sign logic)
Camber_delta = [
    -Camber_s(1) + Camber_d(1);
    -Camber_d(2) - Camber_s(2);
     Camber_d(3) - Camber_s(3);
    -Camber_d(4) - Camber_s(4)
];

% 6. Final Outputs
Camber = Camber_delta + static_camber_4x1;
Camber_gain = Camber_d;
static_camber_visualisation = Camber_s;

end

%% High-Performance Vectorized Helper Function
function Camber_rad = compute_corner_kinematics(zw, UiY, UiZ, LiY, LiZ, UO_Y, LO_Y, TCP_Y, UO_Z_base, LO_Z_base, TCP_Z_base)
    % Apply vertical travel
    UO_Z  = UO_Z_base + zw;
    LO_Z  = LO_Z_base + zw;
    TCP_Z = TCP_Z_base + zw;

    % Slopes of upper & lower arms
    dYU = UO_Y - UiY;
    dYL = LO_Y - LiY;

    % Singularity protection (Replaces previous 0*sign(0) bug)
    dYU = protect_zero(dYU, 1e-6);
    dYL = protect_zero(dYL, 1e-6);

    mU = (UO_Z - UiZ) ./ dYU;
    mL = (LO_Z - LiZ) ./ dYL;

    cU = UiZ - mU .* UiY;
    cL = LiZ - mL .* LiY;

    % Instant Center (IC) Calculation
    den = mU - mL;
    den = protect_zero(den, 1e-6);

    ICy = (cL - cU) ./ den;
    ICz = mU .* ICy + cU;

    % Camber from IC to Contact Patch
    dY = ICy - TCP_Y;
    dZ = ICz - TCP_Z;
    dZ = protect_zero(dZ, 1e-6);

    Camber_rad = -atan(dY ./ dZ);
end

%% Singularity Protection Helper (Coder Safe)
function out = protect_zero(val, tol)
    out = val;
    for i = 1:4
        if abs(out(i)) < tol
            s = sign(out(i));
            if s == 0
                s = 1;
            end
            out(i) = s * tol;
        end
    end
end

== matlab function Vehicle_Model_999_Modular_roll_gradient/Vehicle dynamics/Fx, Fy calculations with grip limit/Slip_angle_calculation/Slip Angles ==
  data: Longitudinal_vel input; slip_angles output; Lateral_vel input; yawrate input; Steer_FL input; Steer_FR input; Par parameter
function slip_angles = fcn(Longitudinal_vel, Lateral_vel, yawrate, Steer_FL, Steer_FR, Par)
%#codegen

    % 1. Geometry Setup
    L = Par.WB;
    T = Par.TW;
    
    % Distance from CG to Axles
    a = L * Par.WD_r;     
    b = L - a;             
    half_T = T / 2;

    % 2. Calculate Velocity Components at Each Corner
    % Kinematic transformation from CG to Hubs
    % Front Left (1)
        Vx_FL = Longitudinal_vel - yawrate * half_T;
        Vy_FL = Lateral_vel + yawrate * a;
    
    % Front Right (2)
        Vx_FR = Longitudinal_vel + yawrate * half_T;
        Vy_FR = Lateral_vel + yawrate * a;
    
    % Rear Left (3)
        Vx_RL = Longitudinal_vel - yawrate * half_T;
        Vy_RL = Lateral_vel - yawrate * b;
    
    % Rear Right (4)
        Vx_RR = Longitudinal_vel + yawrate * half_T;
        Vy_RR = Lateral_vel - yawrate * b;

    % 3. Calculate Velocity Angles (Theta_V)

        Theta_FL = atan2(Vy_FL, max(Vx_FL,0.001));  
        Theta_FR = atan2(Vy_FR, max(Vx_FR,0.001));
        Theta_RL = atan2(Vy_RL, max(Vx_RL,0.001));
        Theta_RR = atan2(Vy_RR, max(Vx_RR,0.001));
    
    % 4. Construct Steering Vector (Delta)
    % Rears are assumed fixed (0 steering)
        Delta = [Steer_FL; Steer_FR; 0; 0];
    
    % Vector of Velocity Angles
        Theta_V = [Theta_FL; Theta_FR; Theta_RL; Theta_RR];

    % 5. Final Calculation
    % Alpha = Delta - Theta_V
        slip_angles = Delta - Theta_V ;
end

== matlab function Vehicle_Model_999_Modular_roll_gradient/Vehicle dynamics/Fx, Fy calculations with grip limit/Slip_ratio_calculation/slip ratios ==
  data: Vx input; Vy input; slip_ratios output; yawrate input; Omega input; Steer_FL input; Steer_FR input; Par parameter
function slip_ratios = fcn(Vx,Vy, yawrate, Omega,Steer_FL,Steer_FR, Par)
%#codegen


    % 1. Constants
    T = Par.TW;
    Re = Par.R0;
    half_T = T / 2;
    a= Par.Lf;
    b=Par.Lr;
    % 2 Yaw Rate Correction (Kinematics)
    
    Vx_FL = Vx - yawrate * half_T;  % Left
    Vx_FR = Vx + yawrate * half_T;  % Right
    Vx_RL = Vx - yawrate * half_T;
    Vx_RR = Vx + yawrate * half_T;
    
    Vx_vec = [Vx_FL; Vx_FR; Vx_RL; Vx_RR];
    
    Vy_FL = Vy + yawrate * a;
    Vy_FR = Vy + yawrate * a;
    Vy_RL = Vy - yawrate * b;
    Vy_RR = Vy - yawrate * b;

    Vy_vec = [Vy_FL; Vy_FR; Vy_RL; Vy_RR];
    Delta = [Steer_FL;Steer_FR;0;0];
    % 3. Slip Angle Correction (Projection)
 
    V_road_plane = Vx_vec .* cos(Delta) + Vy_vec .* sin(Delta);

    % 4. Calculate Wheel Linear Speed
    V_wheel = Omega .* Re;

    % 5. Calculate Slip Ratio
    V_safe_threshold = 0.1; 
    V_ref = max(abs(V_road_plane), V_safe_threshold);
    
    slip_ratios_raw = (V_wheel - V_road_plane) ./ V_ref;
    slip_ratios = slip_ratios_raw;
    % slip_ratios = min(max(slip_ratios_raw,-1),1);
end

== matlab function Vehicle_Model_999_Modular_roll_gradient/Vehicle dynamics/Fx, Fy calculations/Tyre_relaxation/MATLAB Function ==
  data: Fx_ss input; Fx_dot output; Fx_act input; Vx input
function Fx_dot = fcn(Fx_ss, Fx_act, Vx)
    % Fx_ss: Force from Magic Formula block
    % Fx_act: The current integrated force
    % Vx: Longitudinal velocity
    sigma_x = 0.1;
    % Use a small epsilon to avoid division by zero at standstill
    Vx_mod = max(abs(Vx), 0.05); 
    
    % The differential equation
    Fx_dot = (Vx_mod / sigma_x).* (Fx_ss - Fx_act);
end

== matlab function Vehicle_Model_999_Modular_roll_gradient/Vehicle dynamics/Fx, Fy calculations with grip limit/Tyre_relaxation/MATLAB Function ==
  data: Fx_ss input; Fx_dot output; Fx_act input; Vx input
function Fx_dot = fcn(Fx_ss, Fx_act, Vx)
    % Fx_ss: Force from Magic Formula block
    % Fx_act: The current integrated force
    % Vx: Longitudinal velocity
    sigma_x = 0.1;
    % Use a small epsilon to avoid division by zero at standstill
    Vx_mod = max(abs(Vx), 0.05); 
    
    % The differential equation
    Fx_dot = (Vx_mod / sigma_x).* (Fx_ss - Fx_act);
end

== matlab function Vehicle_Model_999_Modular_roll_gradient/Vehicle dynamics/Fx, Fy calculations/Visualise_Fy_B/MATLAB Function ==
  data: Fy_tire input; Fy_B_fl output; Fy_B_fr output; Fy_B_rl output; Fy_B_rr output
function [Fy_B_fl,Fy_B_fr,Fy_B_rl,Fy_B_rr]  = fcn(Fy_tire)

Fy_B_fl = Fy_tire(1);

Fy_B_fr = Fy_tire(2);

Fy_B_rl = Fy_tire(3);

Fy_B_rr = Fy_tire(4);

end

== matlab function Vehicle_Model_999_Modular_roll_gradient/Vehicle dynamics/Fx, Fy calculations with grip limit/Visualise_Fy_B/MATLAB Function ==
  data: Fy_tire input; Fy_B_fl output; Fy_B_fr output; Fy_B_rl output; Fy_B_rr output
function [Fy_B_fl,Fy_B_fr,Fy_B_rl,Fy_B_rr]  = fcn(Fy_tire)

Fy_B_fl = Fy_tire(1);

Fy_B_fr = Fy_tire(2);

Fy_B_rl = Fy_tire(3);

Fy_B_rr = Fy_tire(4);

end

== matlab function Vehicle_Model_999_Modular_roll_gradient/Vehicle dynamics/Fx, Fy calculations with grip limit/Wheel to Vehicle Coordinates ==
  data: Fx_w input; Fx_b output; Fy_w input; Steer_FL input; Steer_FR input; Fy_b output
function [Fx_b, Fy_b] = fcn(Fx_w, Fy_w, Steer_FL, Steer_FR)
%#codegen
% FORCE & MOMENT RESOLVER
    % 1. Construct Steering Vector [FL; FR; RL; RR]
    % Rear steering is assumed to be 0
    Delta = [Steer_FL; Steer_FR; 0; 0];
    
    % 2. Pre-calculate Trig functions (Vectorized)
    c_d = cos(Delta);
    s_d = sin(Delta);
    
    % Longitudinal Body Force:

    Fx_b = Fx_w .* c_d - Fy_w .* s_d;
    
    % Lateral Body Force:
    % Fy_body = Fx_wheel * sin(delta) + Fy_wheel * cos(delta)
    Fy_b = Fx_w .* s_d + Fy_w .* c_d;
    
    % 4. Summation: Total Forces acting on CG
    %B_Fx = sum(Fx_b);
    %B_Fy = sum(Fy_b);
    
end

== matlab function Vehicle_Model_999_Modular_roll_gradient/E-powertrain/Motor/rpm selection for third wheel ==
  data: u input; y output
function y = fcn(u)

y = u(3);

== matlab function Vehicle_Model_999_Modular_roll_gradient/Drivetrain/MATLAB Function ==
  data: T_fl output; T_fr output
function [T_fl,T_fr] = fcn()

T_fl = 0;
T_fr = 0;

== matlab function Vehicle_Model_999_Modular_roll_gradient/E-powertrain/Torque Distribution/Torque Vectoring/MATLAB Function1 ==
  data: u input; y output
function y = fcn(u)
if u > 1e-2 || u < -1e-2
    y = u;
else
    y = 0;
end

== matlab function Vehicle_Model_999_Modular_roll_gradient/Vehicle dynamics/Fx, Fy calculations with grip limit/Grip_limit/MATLAB Function1 ==
  data: Fx input; Fx_new output; Fy input; Dx input; Dy input; s input; Fy_new output
function [Fx_new, Fy_new] = fcn(Fx, Fy, Dx, Dy, s)
    % Initialize outputs
    Fx_new = Fx;
    Fy_new = Fy;
    
    if s > 1
        % 1. Add a tiny protection value (1e-6) to prevent divide-by-zero
        Dx_safe = max(abs(Dx), 1e-3);
        Dy_safe = max(abs(Dy), 1e-3);
        
        % 2. Calculate the grip saturation (eta) for all tires
        eta = sqrt((Fx ./ Dx_safe).^2 + (Fy ./ Dy_safe).^2);
        
        % 3. Find the indices of the tires that are exceeding 100% grip
        over_limit_idx = eta > 1;
        
        % 4. Proportionally scale down ONLY the tires that are slipping
        % This scales the vector perfectly to the edge of the ellipse 
        % without changing the force direction.
        Fx_new(over_limit_idx) = Fx(over_limit_idx) ./ eta(over_limit_idx);
        Fy_new(over_limit_idx) = Fy(over_limit_idx) ./ eta(over_limit_idx);
    end
end

== matlab function Vehicle_Model_999_Modular_roll_gradient/Inputs/steer_input_simulink/MATLAB Function ==
  settings: updateMethod=DISCRETE
  data: X input; delta output; Y input; PSI input; vx input; vy input; path_Y input; path_X input; path_Theta input
function delta = get_steering_command(X, Y, PSI, vx,vy,path_Y, path_X, path_Theta)
    % GET_STEERING_COMMAND Simulink-safe Stanley implementation
   
    %% Parameters
    L_f = 0.78132;          % Pre-multiplied 1.532 * 0.51 for efficiency
    v_eps = 1.0;            % Softening constant to prevent singularity
    v_switch = 5.0;         % Velocity threshold for slip compensation (m/s)
    max_steer = deg2rad(25);% Physical steering limit
    k_stanley = 0;
    %% 1. Sensing (Shift to Front Axle)
    xf = X + L_f * cos(PSI); 
    yf = Y + L_f * sin(PSI);
    
    %% 2. Global Nearest Point Search (Fixed-Size for Simulink)
    % Calculate squared distances to ALL points to maintain fixed array sizes
    dx = path_X - xf;
    dy = path_Y - yf;
    distances = dx.^2 + dy.^2; 
    
    [~, idx_closest] = min(distances);
    Npath = length(path_X);
    
    % %% 3. Path Heading Calculation
    % if Npath <= 1
    %     % Failsafe: If the path is only 1 point, we cannot calculate a slope.
    %     % Default to 0, or you could output an error flag.
    %     path_Theta = 0; 
    % elseif idx_closest < Npath
    %     % Forward difference (standard operation)
    %     path_Theta = atan2(path_X(idx_closest+1) - path_X(idx_closest),path_Y(idx_closest+1) - path_Y(idx_closest));
    % else
    %     % Backward difference (only triggers when exactly on the final point of the track)
    %     path_Theta = atan2(path_X(idx_closest) - path_X(idx_closest-1), path_Y(idx_closest) - path_Y(idx_closest-1));
    % end
    
    %% 4. Error Calculations
    % Crosstrack Error ($e_{ct}$)
    % Cross product mapping ensures right-hand rule sign convention is maintained
    e_ct = (path_Y(idx_closest) - yf)*cos(path_Theta) - (path_X(idx_closest) - xf)*sin(path_Theta);
    
    % Heading Error ($\theta_e$)
    % Wrapped strictly between [-pi, pi]
    theta_e = atan2(sin(path_Theta - PSI), cos(path_Theta - PSI));
    
    %Side_slip calculations:
    beta = atan2(vy,vx);
    
    %% 5. Control Law (Stanley)
    % $\delta = (\theta_e - \beta) + \arctan(k \cdot e_{ct} / (v_x + v_{eps}))$
    delta_raw = (theta_e - beta) + atan2(k_stanley * e_ct, vx + v_eps);
    
    % Apply physical steering limits
    delta = max(min(delta_raw, max_steer), -max_steer);
end

== matlab function Vehicle_Model_999_Modular_roll_gradient/Vehicle dynamics/Fx, Fy calculations with grip limit/MATLAB Function ==
  data: u input; y output
function y = fcn(u)

y = sum(u);
